simulink model "PID_Tracking_control_fin"  (R2023b)
settings: Solver=VariableStepAuto  StartTime=0.0  StopTime=50  RelTol=1e-3
values from neighbouring files (symbols this model uses):
  den_phi = cell2mat(G_t2p_uns.Denominator)    [Rotational_inverted_pendulum.m]
  den_theta = cell2mat(G_ol_uns.Denominator(1,1))    [Rotational_inverted_pendulum.m]
  Kd_phi_v2 = 0    [Rotational_inverted_pendulum.m]
  Kd_theta_v2 = 0.25    [Rotational_inverted_pendulum.m]
  Ki_phi_v2 = 7    [Rotational_inverted_pendulum.m]
  Ki_theta = 0    [Rotational_inverted_pendulum.m]
  Ki_theta_v2 = 0    [Rotational_inverted_pendulum.m]
  Kp_phi_v2 = 0    [Rotational_inverted_pendulum.m]
  Kp_theta = 5    [Rotational_inverted_pendulum.m]
  Kp_theta_v2 = 0.9    [Rotational_inverted_pendulum.m]
  num_phi = cell2mat(G_t2p_uns.Numerator)    [Rotational_inverted_pendulum.m]
  num_theta = cell2mat(G_ol_uns.Numerator(1,1))    [Rotational_inverted_pendulum.m]
  Va_bar = 0    [Rotational_inverted_pendulum.m]
  x1_bar = double(sol.x1)    [Rotational_inverted_pendulum.m]
  x3_bar = 0    [Rotational_inverted_pendulum.m]
libraries: simulink_extras x5, slpidlib x2
settings Model: Creator=Mark  LastModifiedBy=Mark

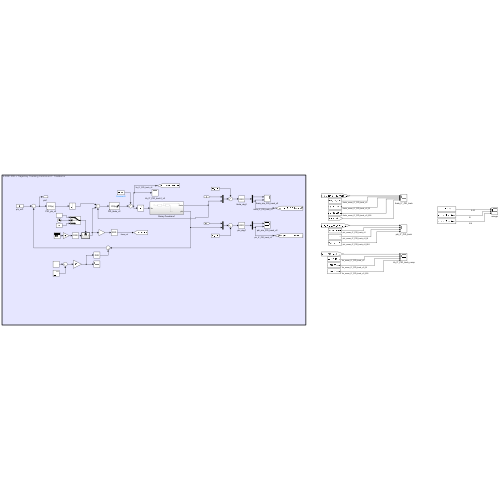
[thumbnail: Simulink's stored preview of the top-level diagram]
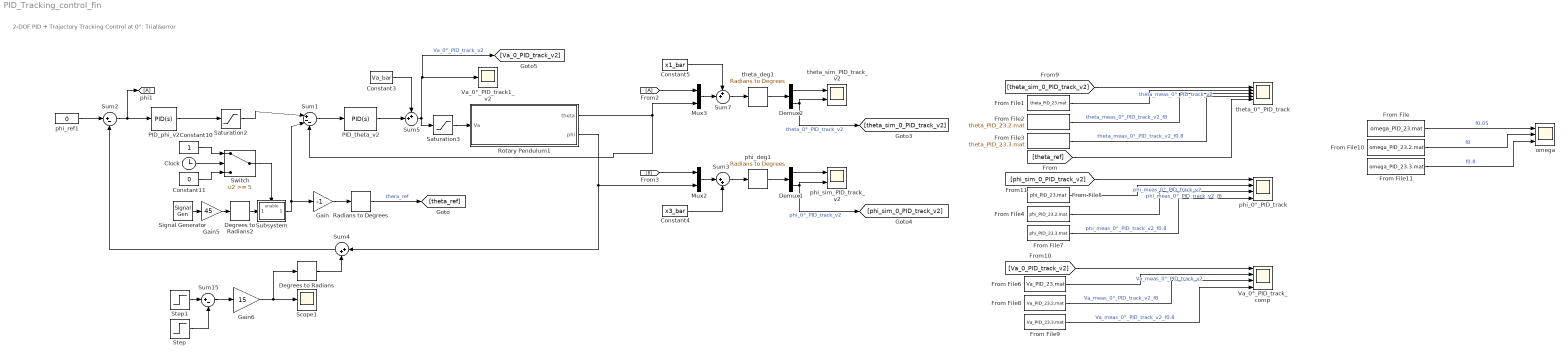
== system PID_Tracking_control_fin ==
  note: 2-DOF PID + Trajectory Tracking Control at 0°: Trial&error
  Clock : Clock
  Constant10 : Constant
  Constant11 : Constant  Value=0
  Constant3 : Constant  Value=Va_bar
  Constant4 : Constant  Value=x3_bar
  Constant5 : Constant  Value=x1_bar
  Degrees to Radians : simulink_extras/Transformations/Degrees to Radians
  Degrees to Radians2 : simulink_extras/Transformations/Degrees to Radians
  Demux1 : Demux  Outputs=2
  Demux2 : Demux  Outputs=2
  From File : FromFile  FileName=omega_PID_23.mat  SampleTime=0
  From File1 : FromFile  FileName=theta_PID_23.mat  SampleTime=0
  From File10 : FromFile  FileName=omega_PID_23.2.mat  SampleTime=0
  From File11 : FromFile  FileName=omega_PID_23.3.mat  SampleTime=0
  From File2 : FromFile  FileName=theta_PID_23.2.mat  SampleTime=0
  From File3 : FromFile  FileName=theta_PID_23.3.mat  SampleTime=0
  From File4 : FromFile  FileName=phi_PID_23.2.mat  SampleTime=0
  From File5 : FromFile  FileName=phi_PID_23.mat  SampleTime=0
  From File6 : FromFile  FileName=Va_PID_23.mat  SampleTime=0
  From File7 : FromFile  FileName=phi_PID_23.3.mat  SampleTime=0
  From File8 : FromFile  FileName=Va_PID_23.2.mat  SampleTime=0
  From File9 : FromFile  FileName=Va_PID_23.3.mat  SampleTime=0
  From2 : From
  Gain : Gain  Gain=-1
  Gain5 : Gain  Gain=45
  Gain6 : Gain  Gain=15
  Mux2 : Mux  Inputs=2
  Mux3 : Mux  Inputs=2
  PID_phi_v2 : slpidlib/PID Controller  Controller=PID  Form=Parallel  TimeDomain=Continuous-time  UseExternalTs=off  SampleTime=-1  IntegratorMethod=Forward Euler  FilterMethod=Forward Euler  ControllerParametersSource=internal  P=Kp_phi_v2  I=Ki_phi_v2  UseKiTs=off  D=Kd_phi_v2  N=100  UseFilter=on  TunerSelectOption=Transfer Function Based (PID Tuner App)  InitialConditionSource=internal  InitialConditionForIntegrator=0  InitialConditionForFilter=0  DifferentiatorICPrevScaledInput=0  ExternalReset=none  TrackingMode=off  Kt=1  LimitOutput=off  SatLimitsSource=internal  UpperSaturationLimit=90  LowerSaturationLimit=-90  LinearizeAsGain=on  AntiWindupMode=none  Kb=1  LimitIntegrator=off  UpperIntegratorSaturationLimit=inf  LowerIntegratorSaturationLimit=-inf  POutMin=[]  POutMax=[]  IOutMin=[]  IOutMax=[]  DOutMin=[]  DOutMax=[]  NOutMin=[]  NOutMax=[]  SumOutMin=[]  SumOutMax=[]  SaturationOutMin=[]  SaturationOutMax=[]  PParamMin=[]  PParamMax=[]  IParamMin=[]  IParamMax=[]  DParamMin=[]  DParamMax=[]  NParamMin=[]  NParamMax=[]  KbParamMin=[]  KbParamMax=[]  KtParamMin=[]  KtParamMax=[]  KbOutMin=[]  KbOutMax=[]  KtOutMin=[]  KtOutMax=[]  IntegratorOutMin=[]  IntegratorOutMax=[]  FilterOutMin=[]  FilterOutMax=[]  SumI1OutMin=[]  SumI1OutMax=[]  SumI2OutMin=[]  SumI2OutMax=[]  SumI3OutMin=[]  SumI3OutMax=[]  SumI4OutMin=[]  SumI4OutMax=[]  SumDOutMin=[]  SumDOutMax=[]  DifferentiatorOutMin=[]  DifferentiatorOutMax=[]  FilterDiffOutCoefMin=[]  FilterDiffOutCoefMax=[]  ReciprocalOutMin=[]  ReciprocalOutMax=[]  SumDenOutMin=[]  SumDenOutMax=[]  SumNumOutMin=[]  SumNumOutMax=[]  DivideOutMin=[]  DivideOutMax=[]  UdiffTsProdOutMin=[]  UdiffTsProdOutMax=[]  NTsProdOutMin=[]  NTsProdOutMax=[]  UintegralTsProdOutMin=[]  UintegralTsProdOutMax=[]  UngainTsProdOutMin=[]  UngainTsProdOutMax=[]  ClampingZeroOutDataTypeStr=Inherit: Inherit via back propagation  ClampingZeroOutMin=[]  ClampingZeroOutMax=[]  FilterDenConstantOutDataTypeStr=Inherit: Inherit via back propagation  FilterDenConstantOutMin=[]  FilterDenConstantOutMax=[]  PCopyOutDataTypeStr=Inherit: Inherit via back propagation  PCopyOutMin=[]  PCopyOutMax=[]  NCopyOutDataTypeStr=Inherit: Inherit via back propagation  NCopyOutMin=[]  NCopyOutMax=[]  IntegratorContinuousStateAttributes=''  IntegratorStateMustResolveToSignalObject=off  IntegratorRTWStateStorageClass=Auto  FilterContinuousStateAttributes=''  FilterStateMustResolveToSignalObject=off  FilterRTWStateStorageClass=Auto  ParallelPVariant=InternalParameters  IdealPVariant=Disabled  IVariant=InternalParameters  DVariant=InternalParameters  IntegratorVariant=Continuous  SatVariant=Disabled  AWVariant=Passthrough  PCopyVariant=Disabled  TRVariant=Disabled  FdbkBlocksVariant=Forward  IdealPFdbkVariant=Disabled  SatFdbkVariant=Disabled  DerivativeFilterVariant=ContFilter  NVariant=InternalParameters  NCopyVariant=Disabled  FilterICVariant=InternalICsFilter  IntegratorICVariant=InternalICs  ExternalResetVariant=Disabled  TRSumVariant=Passthrough  SumFdbkVariant=Disabled  SumVariant=Sum_PID  TsampFilterVariant=InternalTs  TsampNgainVariant=Passthrough  TsampIntegralVariant=Disabled_SignalSpec  ExternalSaturationOutDataTypeStr=Inherit: Same as second input
  PID_theta_v2 : slpidlib/PID Controller  Controller=PID  Form=Parallel  TimeDomain=Continuous-time  UseExternalTs=off  SampleTime=-1  IntegratorMethod=Forward Euler  FilterMethod=Forward Euler  ControllerParametersSource=internal  P=Kp_theta_v2  I=Ki_theta_v2  UseKiTs=off  D=Kd_theta_v2  N=100  UseFilter=on  TunerSelectOption=Transfer Function Based (PID Tuner App)  InitialConditionSource=internal  InitialConditionForIntegrator=0  InitialConditionForFilter=0  DifferentiatorICPrevScaledInput=0  ExternalReset=none  TrackingMode=off  Kt=1  LimitOutput=on  SatLimitsSource=internal  UpperSaturationLimit=10  LowerSaturationLimit=-10  LinearizeAsGain=on  AntiWindupMode=back-calculation  Kb=Ki_theta/Kp_theta  LimitIntegrator=off  UpperIntegratorSaturationLimit=inf  LowerIntegratorSaturationLimit=-inf  POutMin=[]  POutMax=[]  IOutMin=[]  IOutMax=[]  DOutMin=[]  DOutMax=[]  NOutMin=[]  NOutMax=[]  SumOutMin=[]  SumOutMax=[]  SaturationOutMin=[]  SaturationOutMax=[]  PParamMin=[]  PParamMax=[]  IParamMin=[]  IParamMax=[]  DParamMin=[]  DParamMax=[]  NParamMin=[]  NParamMax=[]  KbParamMin=[]  KbParamMax=[]  KtParamMin=[]  KtParamMax=[]  KbOutMin=[]  KbOutMax=[]  KtOutMin=[]  KtOutMax=[]  IntegratorOutMin=[]  IntegratorOutMax=[]  FilterOutMin=[]  FilterOutMax=[]  SumI1OutMin=[]  SumI1OutMax=[]  SumI2OutMin=[]  SumI2OutMax=[]  SumI3OutMin=[]  SumI3OutMax=[]  SumI4OutMin=[]  SumI4OutMax=[]  SumDOutMin=[]  SumDOutMax=[]  DifferentiatorOutMin=[]  DifferentiatorOutMax=[]  FilterDiffOutCoefMin=[]  FilterDiffOutCoefMax=[]  ReciprocalOutMin=[]  ReciprocalOutMax=[]  SumDenOutMin=[]  SumDenOutMax=[]  SumNumOutMin=[]  SumNumOutMax=[]  DivideOutMin=[]  DivideOutMax=[]  UdiffTsProdOutMin=[]  UdiffTsProdOutMax=[]  NTsProdOutMin=[]  NTsProdOutMax=[]  UintegralTsProdOutMin=[]  UintegralTsProdOutMax=[]  UngainTsProdOutMin=[]  UngainTsProdOutMax=[]  ClampingZeroOutDataTypeStr=Inherit: Inherit via back propagation  ClampingZeroOutMin=[]  ClampingZeroOutMax=[]  FilterDenConstantOutDataTypeStr=Inherit: Inherit via back propagation  FilterDenConstantOutMin=[]  FilterDenConstantOutMax=[]  PCopyOutDataTypeStr=Inherit: Inherit via back propagation  PCopyOutMin=[]  PCopyOutMax=[]  NCopyOutDataTypeStr=Inherit: Inherit via back propagation  NCopyOutMin=[]  NCopyOutMax=[]  IntegratorContinuousStateAttributes=''  IntegratorStateMustResolveToSignalObject=off  IntegratorRTWStateStorageClass=Auto  FilterContinuousStateAttributes=''  FilterStateMustResolveToSignalObject=off  FilterRTWStateStorageClass=Auto  ParallelPVariant=InternalParameters  IdealPVariant=Disabled  IVariant=InternalParameters  DVariant=InternalParameters  IntegratorVariant=Continuous  SatVariant=Enabled  AWVariant=BackCalculation  PCopyVariant=Disabled  TRVariant=Disabled  FdbkBlocksVariant=Forward  IdealPFdbkVariant=Disabled  SatFdbkVariant=Disabled  DerivativeFilterVariant=ContFilter  NVariant=InternalParameters  NCopyVariant=Disabled  FilterICVariant=InternalICsFilter  IntegratorICVariant=InternalICs  ExternalResetVariant=Disabled  TRSumVariant=Passthrough  SumFdbkVariant=Disabled  SumVariant=Sum_PID  TsampFilterVariant=InternalTs  TsampNgainVariant=Passthrough  TsampIntegralVariant=Disabled_SignalSpec  ExternalSaturationOutDataTypeStr=Inherit: Same as second input
  Radians to Degrees : simulink_extras/Transformations/Radians to Degrees
  Rotary Pendulum1 : Subsystem
  Saturation2 : Saturate  UpperLimit=pi/2  LowerLimit=-pi/2
  Saturation3 : Saturate  UpperLimit=10  LowerLimit=-10
  Scope1 : Scope
  Signal Generator : SignalGenerator  Frequency=8
  Step : Step  Time=20.05  SampleTime=0
  Step1 : Step  Time=20  SampleTime=0
  Subsystem : Subsystem
  Sum1 : Sum  Inputs=|+--
  Sum15 : Sum  Inputs=|+-
  Sum2 : Sum  Inputs=|+-
  Sum3 : Sum  Inputs=|++
  Sum4 : Sum  Inputs=|++
  Sum5 : Sum  Inputs=++|
  Sum7 : Sum  Inputs=++|
  Switch : Switch  Threshold=5  SaturateOnIntegerOverflow=off  InputSameDT=off
  Va_0°_PID_track1_v2 : Scope
  Va_0°_PID_track_comp : Scope  NumInputPorts=4
  omega : Scope  NumInputPorts=3
  phi1 : Goto
  phi_0°_PID_track : Scope  NumInputPorts=4
  phi_deg1 : simulink_extras/Transformations/Radians to Degrees
  phi_ref1 : Constant  Value=0
  phi_sim_PID_track_v2 : Scope  NumInputPorts=2
  theta_0°_PID_track : Scope  NumInputPorts=5
  theta_deg1 : simulink_extras/Transformations/Radians to Degrees
  theta_sim_PID_track_v2 : Scope  NumInputPorts=2
  wires:
  Sum15/1 -> Gain6/1
  Gain6/1 -> Scope1/1, Degrees to Radians/1
  Step/1 -> Sum15/2
  Step1/1 -> Sum15/1
  theta_deg1/1 -> Demux2/1
  phi_ref1/1 -> Sum2/1
  Mux2/1 -> Sum3/1
  PID_theta_v2/1 -> Sum5/2
  Rotary Pendulum1/1(theta) -> Sum1/3, Mux3/2
  Saturation2/1 -> Sum1/1
  Sum7/1 -> theta_deg1/1
  Demux2/1 -> theta_sim_PID_track_v2/1
  Saturation3/1 -> Rotary Pendulum1/1(Va)
  Constant4/1 -> Sum3/2
  Sum5/1 -> Saturation3/1, [Va_0_PID_track_v2], Va_0°_PID_track1_v2/1  "Va_0°_PID_track_v2"
  PID_phi_v2/1 -> Saturation2/1
  Demux2/2 -> [theta_sim_0_PID_track_v2], theta_sim_PID_track_v2/2  "theta_0°_PID_track_v2"
  Constant5/1 -> Sum7/1
  phi_deg1/1 -> Demux1/1
  Constant3/1 -> Sum5/1
  Mux3/1 -> Sum7/2
  Rotary Pendulum1/2(phi) -> Sum4/1, Mux2/2
  [B] -> Mux2/1
  Sum4/1 -> Sum2/2
  Demux1/2 -> [phi_sim_0_PID_track_v2], phi_sim_PID_track_v2/2  "phi_0°_PID_track_v2"
  Demux1/1 -> phi_sim_PID_track_v2/1
  Sum2/1 -> PID_phi_v2/1, phi1/1
  From2/1 -> Mux3/1
  Sum3/1 -> phi_deg1/1
  Sum1/1 -> PID_theta_v2/1
  [Va_0_PID_track_v2] -> Va_0°_PID_track_comp/1
  [phi_sim_0_PID_track_v2] -> phi_0°_PID_track/1
  [theta_sim_0_PID_track_v2] -> theta_0°_PID_track/1
  From File5/1 -> phi_0°_PID_track/2  "phi_meas_0°_PID_track_v2"
  From File6/1 -> Va_0°_PID_track_comp/2  "Va_meas_0°_PID_track_v2"
  From File1/1 -> theta_0°_PID_track/2  "theta_meas_0°_PID_track_v2"
  Degrees to Radians/1 -> Sum4/2
  Subsystem/1(Out1) -> Gain/1, Sum1/2
  Switch/1 -> Subsystem/Enable
  Signal Generator/1 -> Gain5/1
  Constant10/1 -> Switch/1
  Constant11/1 -> Switch/3
  Clock/1 -> Switch/2
  Gain5/1 -> Degrees to Radians2/1
  Degrees to Radians2/1 -> Subsystem/1(In1)
  From File/1 -> omega/1  "f0.05"
  From File2/1 -> theta_0°_PID_track/3  "theta_meas_0°_PID_track_v2_f8"
  From File3/1 -> theta_0°_PID_track/4  "theta_meas_0°_PID_track_v2_f0.8"
  From File4/1 -> phi_0°_PID_track/3  "phi_meas_0°_PID_track_v2_f8"
  From File7/1 -> phi_0°_PID_track/4  "phi_meas_0°_PID_track_v2_f0.8"
  From File8/1 -> Va_0°_PID_track_comp/3  "Va_meas_0°_PID_track_v2_f8"
  From File9/1 -> Va_0°_PID_track_comp/4  "Va_meas_0°_PID_track_v2_f0.8"
  From File10/1 -> omega/2  "f8"
  From File11/1 -> omega/3  "f0.8"
  [theta_ref] -> theta_0°_PID_track/5
  Radians to Degrees/1 -> [theta_ref]  "thera_ref"
  Gain/1 -> Radians to Degrees/1

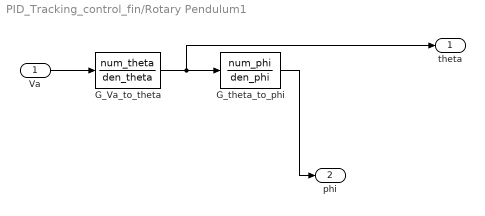
== system PID_Tracking_control_fin/Rotary Pendulum1 ==
  Va : Inport
  G_Va_to_theta : TransferFcn  Numerator=num_theta  Denominator=den_theta
  G_theta_to_phi : TransferFcn  Numerator=num_phi  Denominator=den_phi
  theta : Outport
  phi : Outport  Port=2
  wires:
  G_theta_to_phi/1 -> phi/1
  G_Va_to_theta/1 -> theta/1, G_theta_to_phi/1
  Va/1 -> G_Va_to_theta/1

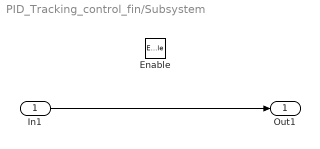
== system PID_Tracking_control_fin/Subsystem ==
  In1 : Inport
  Enable : EnablePort
  Out1 : Outport
  wires:
  In1/1 -> Out1/1
